simulink model "PD"  (R2019b)
settings: Solver=VariableStepAuto  StartTime=0.0  StopTime=10.0  RelTol=1e-3
undefined symbols (not defined in the file): parameter
settings Model: Creator=Giga  LastModifiedBy=Giga

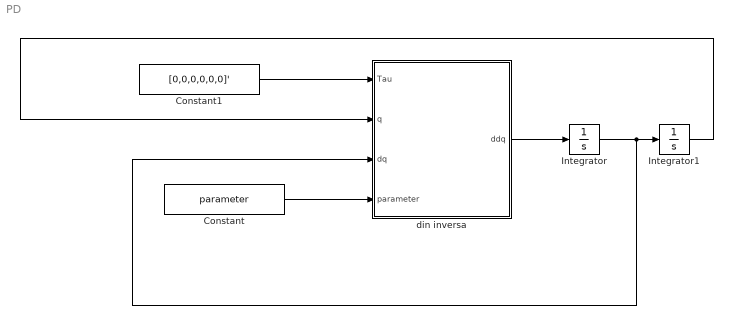
== system PD ==
  Constant : Constant  Value=parameter
  Constant1 : Constant  Value=[0,0,0,0,0,0]'
  Integrator : Integrator  InitialCondition=[0,0,0,0,0,0]'
  Integrator1 : Integrator  InitialCondition=[0,0,0,0,0,0]'
  din inversa : MATLAB Function  TreatAsAtomicUnit=on
  wires:
  din inversa/1(ddq) -> Integrator/1
  Integrator/1 -> din inversa/3(dq), Integrator1/1
  Constant/1 -> din inversa/4(parameter)
  Integrator1/1 -> din inversa/2(q)
  Constant1/1 -> din inversa/1(Tau)

== matlab function PD/din inversa ==
  data: Tau input; ddq output; q input; dq input; parameter input
function ddq = dinI(Tau,q,dq,parameter)

    B = B_f(parameter,q,dq);
    C = C_f(parameter,q,dq)
    G = G_f(parameter,q,dq);
    
    ddq = B\(Tau-C*dq-G);
    
end
